simulink model "pet_thirsty"  (R2023a)
settings: Solver=VariableStepAuto  StartTime=0.0  StopTime=24.0  RelTol=1e-3
settings Model: Creator=laurabryant  LastModifiedBy=laurabryant

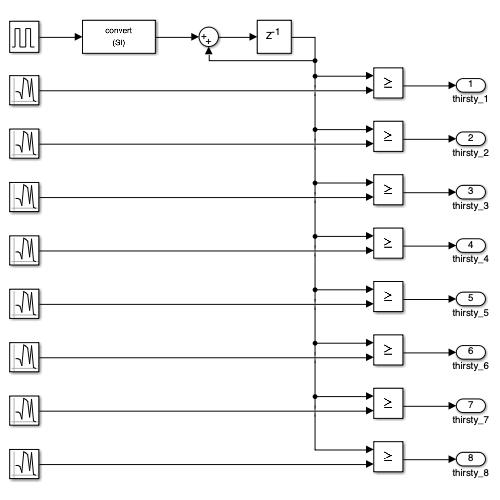
[thumbnail: Simulink's stored preview of the top-level diagram]
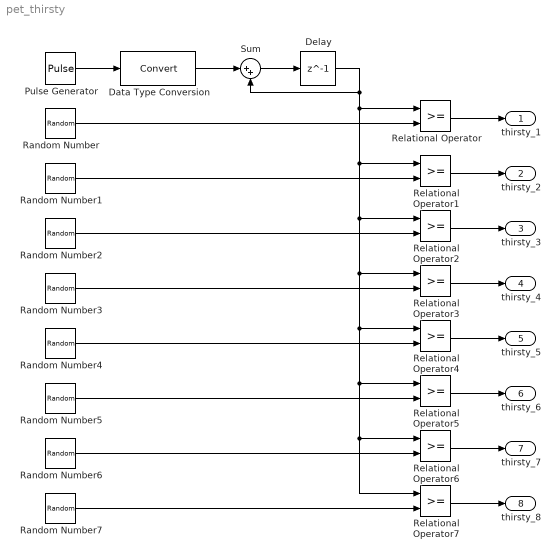
== system pet_thirsty ==
  Data Type Conversion : DataTypeConversion  OutMin=0  OutMax=1  ConvertRealWorld=Stored Integer (SI)  RndMeth=Nearest  SaturateOnIntegerOverflow=off
  Delay : Delay  DelayLength=1  InitialCondition=0  SampleTime=1
  Pulse Generator : DiscretePulseGenerator  PulseType=Time based  Period=1  PulseWidth=5
  Random Number : RandomNumber  Mean=3  SampleTime=48
  Random Number1 : RandomNumber  Mean=9  Seed=1  SampleTime=48
  Random Number2 : RandomNumber  Mean=15  Seed=2  SampleTime=48
  Random Number3 : RandomNumber  Mean=21  Seed=3  SampleTime=48
  Random Number4 : RandomNumber  Mean=27  Seed=4  SampleTime=48
  Random Number5 : RandomNumber  Mean=33  Seed=5  SampleTime=48
  Random Number6 : RandomNumber  Mean=39  Seed=6  SampleTime=48
  Random Number7 : RandomNumber  Mean=45  Seed=7  SampleTime=48
  Relational Operator{,1..7} (8 alike) : RelationalOperator  OutDataTypeStr=boolean  RndMeth=Simplest  InputSameDT=off
  Sum : Sum  Inputs=|++
  thirsty_1 : Outport
  thirsty_2 : Outport  Port=2
  thirsty_3 : Outport  Port=3
  thirsty_4 : Outport  Port=4
  thirsty_5 : Outport  Port=5
  thirsty_6 : Outport  Port=6
  thirsty_7 : Outport  Port=7
  thirsty_8 : Outport  Port=8
  wires:
  Relational Operator2/1 -> thirsty_3/1
  Relational Operator/1 -> thirsty_1/1
  Random Number/1 -> Relational Operator/2
  Random Number2/1 -> Relational Operator2/2
  Random Number1/1 -> Relational Operator1/2
  Sum/1 -> Delay/1
  Relational Operator1/1 -> thirsty_2/1
  Data Type Conversion/1 -> Sum/1
  Pulse Generator/1 -> Data Type Conversion/1
  Random Number3/1 -> Relational Operator3/2
  Random Number4/1 -> Relational Operator4/2
  Random Number5/1 -> Relational Operator5/2
  Relational Operator3/1 -> thirsty_4/1
  Relational Operator4/1 -> thirsty_5/1
  Relational Operator5/1 -> thirsty_6/1
  Random Number6/1 -> Relational Operator6/2
  Relational Operator6/1 -> thirsty_7/1
  Delay/1 -> Relational Operator/1, Relational Operator6/1, Relational Operator7/1, Relational Operator5/1, Relational Operator4/1, Relational Operator3/1, Relational Operator2/1, Relational Operator1/1, Sum/2
  Random Number7/1 -> Relational Operator7/2
  Relational Operator7/1 -> thirsty_8/1
